simulink model "IM_ScalarCtl_adv_exercise"  (R2013b)
settings: Solver=ode45  StartTime=0.0  StopTime=3  MaxStep=1e-3  RelTol=1e-6
values from neighbouring files (symbols this model uses):
  fR = fn    (= 50)    [im_data.m]
  freq_sn = (ns-nn)/ns*fn    (= 2.33333333333)    [im_data.m]
  IactRated = In*sqrt(2)*PF    [im_data.m]
  J = jm    (= 0.0069)    [im_data.m]
  Lm = 235.0e-3    (= 0.235)    [im_data.m]
  Lr = Lm + Ldr    (= 0.24729)    [im_data.m]
  Ls = Lm + Lds    (= 0.2442)    [im_data.m]
  p = 2.0    (= 2)    [im_data.m]
  Rr = 2.32    [im_data.m]
  Rs = 3.67*1.5    (= 5.505)    [im_data.m]
  Vs0 = Un    (= 220)    [im_data.m]
libraries: powerlib_meascontrol x2, simulink x1
settings Model: Creator=unnikrishnan  LastModifiedBy=Fitim k
settings DataIOCC: SignalLoggingSaveFormat=ModelDataLogs
settings OptimizationCC: InitFltsAndDblsToZero=on
settings DebuggingCC: SaveWithParameterizedLinksMsg=none  SignalResolutionControl=TryResolveAllWithWarning  MultiTaskDSMMsg=warning  MultiTaskCondExecSysMsg=none  FcnCallInpInsideContextMsg=UseLocalSettings  StateNameClashWarn=warning
settings RTWCC: IncludeERTFirstTime=on
settings GRTTargetCC: TargetFcnLib=ansi_tfl_tmw.mat  CombineOutputUpdateFcns=off  GRTInterface=on

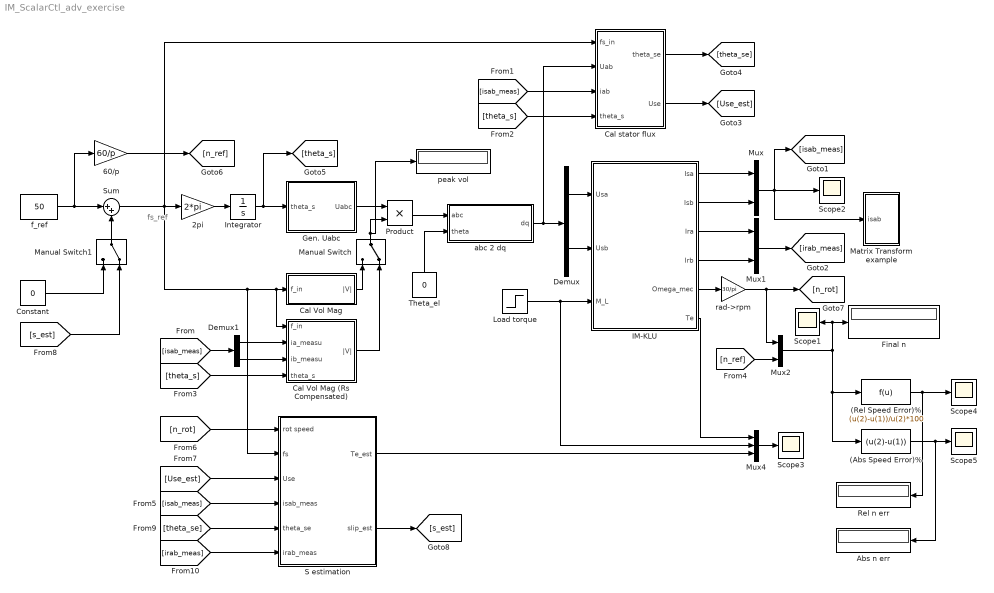
== system IM_ScalarCtl_adv_exercise ==
  note: fs_ref
  (Abs Speed Error)% : Fcn  Expr=(u(2)-u(1))
  (Rel Speed Error)% : Fcn  Expr=(u(2)-u(1))/u(2)*100
  2pi : Gain  Gain=2*pi
  60/p : Gain  Gain=60/p
  Abs n err : Display
  Cal Vol Mag : Subsystem
  Cal Vol Mag (Rs Compensated) : Subsystem
  Cal stator flux : Subsystem
  Constant : Constant  Value=0
  Demux : Demux  Outputs=2
  Demux1 : Demux  Outputs=2
  Final n : Display
  Gen. Uabc : Subsystem
  IM-KLU : Subsystem  mask(IM parameters){ms=3, pb=p, J=J, Lm=Lm, Lr=Lr, Ls=Ls, Rr=Rr, Rs=Rs}
      mask prompts: ms "number of pases"; pb "pole pairs"
  Integrator : Integrator
  Load torque : Step  After=14.6912  SampleTime=0
  Manual Switch : ManualSwitch  CurrentSetting=0
  Manual Switch1 : ManualSwitch  CurrentSetting=0
  Matrix Transform example : Subsystem
  Mux : Mux  Inputs=2
  Mux1 : Mux  Inputs=2
  Mux2 : Mux  Inputs=2
  Mux4 : Mux  Inputs=3
  Product : Product  RndMeth=Zero
  Rel n err : Display
  S estimation : Subsystem
  Scope{1..5} (5 alike) : Scope
      Scope1 settings: TimeRange=0.2881844380403459  YMin=1435  YMax=1500  SaveName=ScopeData2
      Scope2 settings: YMin=-7  YMax=7
      Scope3 settings: YMin=-2.5  YMax=25
      Scope4 settings: TimeRange=3  YMin=5.02075  YMax=5.021  SaveName=ScopeData3
      Scope5 settings: TimeRange=0.2881844380403459  YMin=0  YMax=1197.83  SaveName=ScopeData4
  Sum : Sum  Inputs=|++
  Theta_el : Constant  Value=0
  abc 2 dq : Subsystem
  f_ref : Constant  Value=50
  peak vol : Display
  rad->rpm : Gain  Gain=30/pi  SaturateOnIntegerOverflow=on  OutDataTypeStr=Inherit: Same as input  ParamDataTypeStr=Inherit: Same as input
  wires:
  f_ref/1 -> Sum/1, 60/p/1
  Constant/1 -> Manual Switch1/1
  Manual Switch1/1 -> Sum/2
  2pi/1 -> Integrator/1
  Integrator/1 -> Gen. Uabc/1(theta_s), [theta_s]
  Theta_el/1 -> abc 2 dq/2(theta)
  Product/1 -> abc 2 dq/1(abc)
  Gen. Uabc/1(Uabc) -> Product/1
  abc 2 dq/1(dq) -> Demux/1, Cal stator flux/2(Uab)
  Demux/1 -> IM-KLU/1(Usa)
  Demux/2 -> IM-KLU/2(Usb)
  Load torque/1 -> IM-KLU/3(M_L), Mux4/2
  IM-KLU/1(Isa) -> Mux/1
  IM-KLU/2(Isb) -> Mux/2
  Mux/1 -> Scope2/1, [isab_meas], Matrix Transform example/1(isab)
  IM-KLU/3(Ira) -> Mux1/1
  IM-KLU/4(Irb) -> Mux1/2
  Mux1/1 -> [irab_meas]
  Mux4/1 -> Scope3/1
  IM-KLU/6(Te) -> Mux4/1
  Mux2/1 -> (Rel Speed Error)%/1, (Abs Speed Error)%/1, Final n/1, Scope1/1
  (Rel Speed Error)%/1 -> Scope4/1, Rel n err/1
  (Abs Speed Error)%/1 -> Scope5/1, Abs n err/1
  IM-KLU/5(Omega_mec) -> rad->rpm/1
  rad->rpm/1 -> Mux2/1, [n_rot]
  Sum/1 -> 2pi/1, Cal stator flux/1(fs_in), S estimation/2(fs), Cal Vol Mag (Rs Compensated)/1(f_in), Cal Vol Mag/1(f_in)
  Demux1/1 -> Cal Vol Mag (Rs Compensated)/2(ia_measu)
  Demux1/2 -> Cal Vol Mag (Rs Compensated)/3(ib_measu)
  [isab_meas] -> Demux1/1
  Cal stator flux/1(theta_se) -> [theta_se]
  Cal stator flux/2(Use) -> [Use_est]
  [isab_meas] -> Cal stator flux/3(iab)
  [theta_s] -> Cal stator flux/4(theta_s)
  [theta_s] -> Cal Vol Mag (Rs Compensated)/4(theta_s)
  60/p/1 -> [n_ref]
  [n_ref] -> Mux2/2
  [n_rot] -> S estimation/1(rot speed)
  [Use_est] -> S estimation/3(Use)
  [isab_meas] -> S estimation/4(isab_meas)
  S estimation/2(slip_est) -> [s_est]
  [s_est] -> Manual Switch1/2
  [theta_se] -> S estimation/5(theta_se)
  [irab_meas] -> S estimation/6(irab_meas)
  Manual Switch/1 -> Product/2, peak vol/1
  Cal Vol Mag/1(|V|) -> Manual Switch/1
  Cal Vol Mag (Rs Compensated)/1(|V|) -> Manual Switch/2
  S estimation/1(Te_est) -> Mux4/3

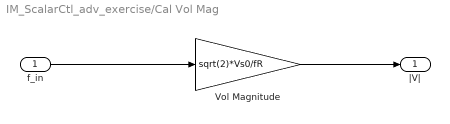
== system IM_ScalarCtl_adv_exercise/Cal Vol Mag ==
  f_in : Inport
  Vol Magnitude : Gain  Gain=sqrt(2)*Vs0/fR
  |V| : Outport
  wires:
  f_in/1 -> Vol Magnitude/1
  Vol Magnitude/1 -> |V|/1

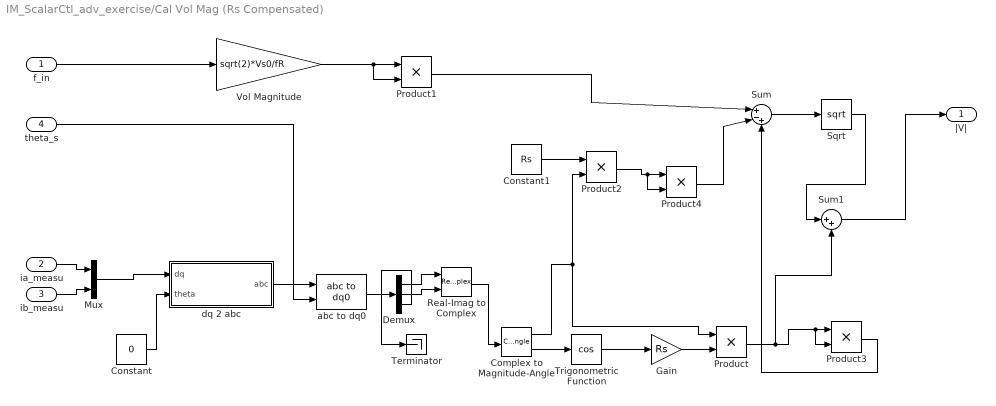
== system IM_ScalarCtl_adv_exercise/Cal Vol Mag (Rs Compensated) ==
  f_in : Inport
  ia_measu : Inport  Port=2
  ib_measu : Inport  Port=3
  theta_s : Inport  Port=4
  Complex to Magnitude-Angle : ComplexToMagnitudeAngle
  Constant : Constant  Value=0
  Constant1 : Constant  Value=Rs
  Demux : Demux  Outputs=3
  Gain : Gain  Gain=Rs
  Mux : Mux  Inputs=2
  Product{,1..4} (5 alike) : Product
  Real-Imag to Complex : RealImagToComplex
  Sqrt : Sqrt  SaturateOnIntegerOverflow=on
  Sum : Sum  Inputs=|+-+
  Sum1 : Sum  Inputs=|++
  Terminator : Terminator
  Trigonometric Function : Trigonometry  Operator=cos
  Vol Magnitude : Gain  Gain=sqrt(2)*Vs0/fR
  abc to dq0 : powerlib_meascontrol/Transformations/abc to dq0  Alignment=Aligned with phase A axis
  dq 2 abc : Subsystem
  |V| : Outport
  wires:
  ib_measu/1 -> Mux/2
  ia_measu/1 -> Mux/1
  Constant/1 -> dq 2 abc/2(theta)
  dq 2 abc/1(abc) -> abc to dq0/1
  theta_s/1 -> abc to dq0/2
  abc to dq0/1 -> Demux/1
  Demux/1 -> Real-Imag to Complex/1
  Demux/2 -> Real-Imag to Complex/2
  Real-Imag to Complex/1 -> Complex to Magnitude-Angle/1
  Demux/3 -> Terminator/1
  f_in/1 -> Vol Magnitude/1
  Complex to Magnitude-Angle/2 -> Trigonometric Function/1
  Trigonometric Function/1 -> Gain/1
  Complex to Magnitude-Angle/1 -> Product/1, Product2/2
  Vol Magnitude/1 -> Product1/2, Product1/1
  Gain/1 -> Product/2
  Constant1/1 -> Product2/1
  Product/1 -> Sum1/2, Product3/2, Product3/1
  Product3/1 -> Sum/3
  Product2/1 -> Product4/2, Product4/1
  Product1/1 -> Sum/1
  Product4/1 -> Sum/2
  Sum/1 -> Sqrt/1
  Sqrt/1 -> Sum1/1
  Sum1/1 -> |V|/1
  Mux/1 -> dq 2 abc/1(dq)

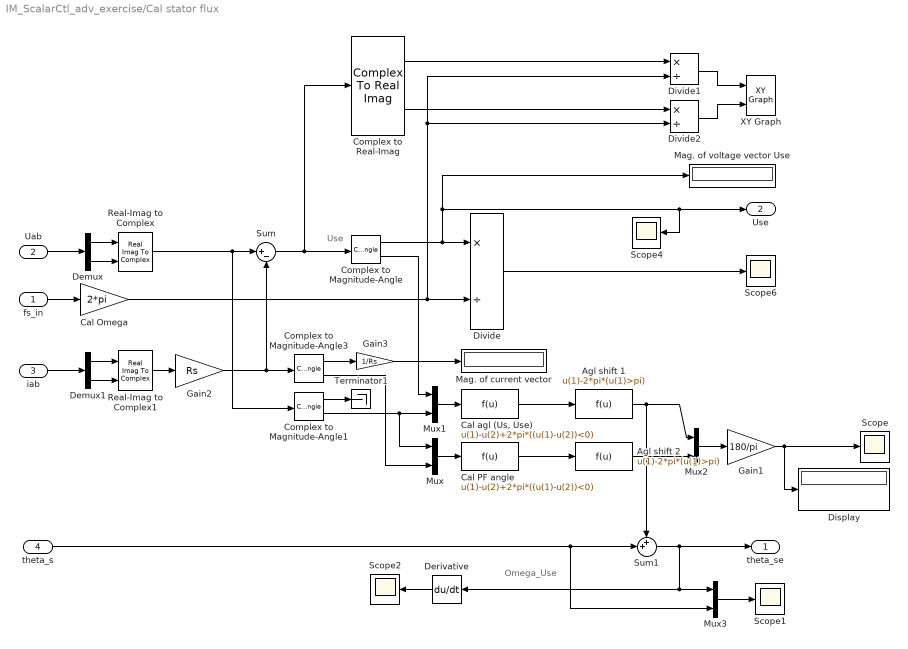
== system IM_ScalarCtl_adv_exercise/Cal stator flux ==
  note: Use
  note: Omega_Use
  fs_in : Inport
  Uab : Inport  Port=2
  iab : Inport  Port=3
  theta_s : Inport  Port=4
  Agl shift 1 : Fcn  Expr=u(1)-2*pi*(u(1)>pi)
  Agl shift 2 : Fcn  Expr=u(1)-2*pi*(u(1)>pi)
  Cal Omega : Gain  Gain=2*pi
  Cal PF angle : Fcn  Expr=u(1)-u(2)+2*pi*((u(1)-u(2))<0)
  "Cal agl (Us, Use)" : Fcn  Expr=u(1)-u(2)+2*pi*((u(1)-u(2))<0)
  Complex to Magnitude-Angle : ComplexToMagnitudeAngle
  Complex to Magnitude-Angle1 : ComplexToMagnitudeAngle
  Complex to Magnitude-Angle3 : ComplexToMagnitudeAngle
  Complex to Real-Imag : ComplexToRealImag
  Demux : Demux  Outputs=2
  Demux1 : Demux  Outputs=2
  Derivative : Derivative
  Display : Display
  Divide : Product  Inputs=*/
  Divide1 : Product  Inputs=*/
  Divide2 : Product  Inputs=*/
  Gain1 : Gain  Gain=180/pi
  Gain2 : Gain  Gain=Rs
  Gain3 : Gain  Gain=1/Rs
  Mag. of current vector : Display
  Mag. of voltage vector Use : Display
  Mux{,1..3} (4 alike) : Mux  Inputs=2
  Real-Imag to Complex : RealImagToComplex
  Real-Imag to Complex1 : RealImagToComplex
  Scope{,1..2,4,6} (5 alike) : Scope
      Scope settings: YMin=-90  YMax=140  SaveName=ScopeData9
      Scope1 settings: YMin=-90  YMax=140  SaveName=ScopeData5
      Scope2 settings: YMin=-90  YMax=140  SaveName=ScopeData10
      Scope4 settings: TimeRange=0.2881844380403459  YMin=158.3  YMax=159.4  SaveName=ScopeData21
      Scope6 settings: TimeRange=0.2881844380403459  YMin=0.940831  YMax=1.03987  SaveName=ScopeData6
  Sum : Sum  Inputs=|+-
  Sum1 : Sum  Inputs=++|
  Terminator1 : Terminator
  XY Graph : simulink/Sinks/XY Graph  xmin=-1.5  xmax=1.5  ymin=-1.5  ymax=1.5  st=-1
  theta_se : Outport
  Use : Outport  Port=2
  wires:
  Complex to Magnitude-Angle/1 -> Divide/1, Mag. of voltage vector Use/1, Use/1, Scope4/1
  Cal Omega/1 -> Divide/2, Divide2/2, Divide1/2
  fs_in/1 -> Cal Omega/1
  Complex to Real-Imag/1 -> Divide1/1
  Complex to Real-Imag/2 -> Divide2/1
  Divide1/1 -> XY Graph/1
  Divide2/1 -> XY Graph/2
  Mux/1 -> Cal PF angle/1
  Gain1/1 -> Display/1, Scope/1
  Mux1/1 -> "Cal agl (Us, Use)"/1
  Mux2/1 -> Gain1/1
  Cal PF angle/1 -> Agl shift 2/1
  "Cal agl (Us, Use)"/1 -> Agl shift 1/1
  Divide/1 -> Scope6/1
  Gain2/1 -> Sum/2, Complex to Magnitude-Angle3/1
  Sum/1 -> Complex to Magnitude-Angle/1, Complex to Real-Imag/1
  Complex to Magnitude-Angle1/1 -> Terminator1/1
  Complex to Magnitude-Angle1/2 -> Mux/1, Mux1/2
  Complex to Magnitude-Angle3/1 -> Gain3/1
  Complex to Magnitude-Angle3/2 -> Mux/2
  Agl shift 1/1 -> Mux2/1, Sum1/1
  Agl shift 2/1 -> Mux2/2
  theta_s/1 -> Sum1/2, Mux3/2
  Sum1/1 -> theta_se/1, Mux3/1, Derivative/1
  Uab/1 -> Demux/1
  Demux/1 -> Real-Imag to Complex/1
  Demux/2 -> Real-Imag to Complex/2
  Real-Imag to Complex/1 -> Sum/1, Complex to Magnitude-Angle1/1
  Demux1/1 -> Real-Imag to Complex1/1
  iab/1 -> Demux1/1
  Real-Imag to Complex1/1 -> Gain2/1
  Demux1/2 -> Real-Imag to Complex1/2
  Mux3/1 -> Scope1/1
  Complex to Magnitude-Angle/2 -> Mux1/1
  Derivative/1 -> Scope2/1
  Gain3/1 -> Mag. of current vector/1

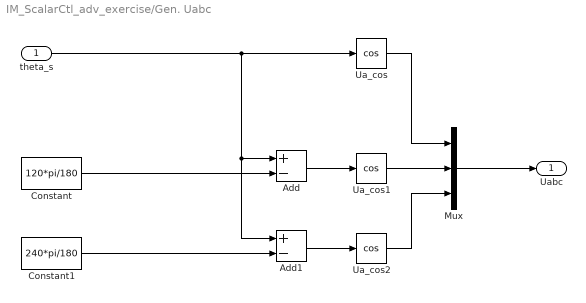
== system IM_ScalarCtl_adv_exercise/Gen. Uabc ==
  theta_s : Inport
  Add : Sum  Inputs=+-
  Add1 : Sum  Inputs=+-
  Constant : Constant  Value=120*pi/180
  Constant1 : Constant  Value=240*pi/180
  Mux : Mux  Inputs=3
  Ua_cos : Trigonometry  Operator=cos
  Ua_cos1 : Trigonometry  Operator=cos
  Ua_cos2 : Trigonometry  Operator=cos
  Uabc : Outport
  wires:
  Constant/1 -> Add/2
  Constant1/1 -> Add1/2
  theta_s/1 -> Ua_cos/1, Add/1, Add1/1
  Add/1 -> Ua_cos1/1
  Add1/1 -> Ua_cos2/1
  Ua_cos/1 -> Mux/1
  Ua_cos1/1 -> Mux/2
  Ua_cos2/1 -> Mux/3
  Mux/1 -> Uabc/1

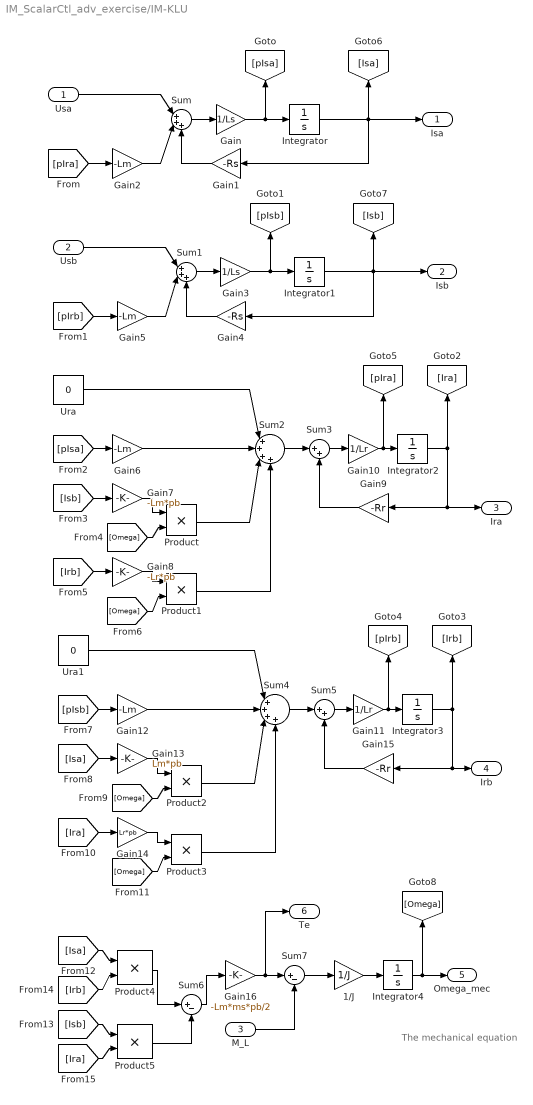
== system IM_ScalarCtl_adv_exercise/IM-KLU ==
  note: The mechanical equation
  Usa : Inport
  Usb : Inport  Port=2
  M_L : Inport  Port=3
  1/J : Gain  Gain=1/J  SaturateOnIntegerOverflow=on  OutDataTypeStr=Inherit: Same as input  ParamDataTypeStr=Inherit: Same as input
  Gain : Gain  Gain=1/Ls  SaturateOnIntegerOverflow=on  OutDataTypeStr=Inherit: Same as input  ParamDataTypeStr=Inherit: Same as input
  Gain1 : Gain  Gain=-Rs  SaturateOnIntegerOverflow=on  OutDataTypeStr=Inherit: Same as input  ParamDataTypeStr=Inherit: Same as input
  Gain10 : Gain  Gain=1/Lr  SaturateOnIntegerOverflow=on  OutDataTypeStr=Inherit: Same as input  ParamDataTypeStr=Inherit: Same as input
  Gain11 : Gain  Gain=1/Lr  SaturateOnIntegerOverflow=on  OutDataTypeStr=Inherit: Same as input  ParamDataTypeStr=Inherit: Same as input
  Gain{2,5..6,12} (4 alike) : Gain  Gain=-Lm  SaturateOnIntegerOverflow=on  OutDataTypeStr=Inherit: Same as input  ParamDataTypeStr=Inherit: Same as input
  Gain13 : Gain  Gain=Lm*pb  SaturateOnIntegerOverflow=on  OutDataTypeStr=Inherit: Same as input  ParamDataTypeStr=Inherit: Same as input
  Gain14 : Gain  Gain=Lr*pb  SaturateOnIntegerOverflow=on  OutDataTypeStr=Inherit: Same as input  ParamDataTypeStr=Inherit: Same as input
  Gain15 : Gain  Gain=-Rr  SaturateOnIntegerOverflow=on  OutDataTypeStr=Inherit: Same as input  ParamDataTypeStr=Inherit: Same as input
  Gain16 : Gain  Gain=-Lm*ms*pb/2  SaturateOnIntegerOverflow=on  OutDataTypeStr=Inherit: Same as input  ParamDataTypeStr=Inherit: Same as input
  Gain3 : Gain  Gain=1/Ls  SaturateOnIntegerOverflow=on  OutDataTypeStr=Inherit: Same as input  ParamDataTypeStr=Inherit: Same as input
  Gain4 : Gain  Gain=-Rs  SaturateOnIntegerOverflow=on  OutDataTypeStr=Inherit: Same as input  ParamDataTypeStr=Inherit: Same as input
  Gain7 : Gain  Gain=-Lm*pb  SaturateOnIntegerOverflow=on  OutDataTypeStr=Inherit: Same as input  ParamDataTypeStr=Inherit: Same as input
  Gain8 : Gain  Gain=-Lr*pb  SaturateOnIntegerOverflow=on  OutDataTypeStr=Inherit: Same as input  ParamDataTypeStr=Inherit: Same as input
  Gain9 : Gain  Gain=-Rr  SaturateOnIntegerOverflow=on  OutDataTypeStr=Inherit: Same as input  ParamDataTypeStr=Inherit: Same as input
  Integrator{,1..4} (5 alike) : Integrator
  Product{,1..5} (6 alike) : Product  SaturateOnIntegerOverflow=on  RndMeth=Zero  InputSameDT=on  OutDataTypeStr=Inherit: Same as first input
  Sum : Sum  Inputs=|+++  SaturateOnIntegerOverflow=on  InputSameDT=on  OutDataTypeStr=Inherit: Same as first input
  Sum1 : Sum  Inputs=|+++  SaturateOnIntegerOverflow=on  InputSameDT=on  OutDataTypeStr=Inherit: Same as first input
  Sum2 : Sum  Inputs=|++++  SaturateOnIntegerOverflow=on  InputSameDT=on  OutDataTypeStr=Inherit: Same as first input
  Sum3 : Sum  Inputs=|++  SaturateOnIntegerOverflow=on  InputSameDT=on  OutDataTypeStr=Inherit: Same as first input
  Sum4 : Sum  Inputs=|++++  SaturateOnIntegerOverflow=on  InputSameDT=on  OutDataTypeStr=Inherit: Same as first input
  Sum5 : Sum  Inputs=|++  SaturateOnIntegerOverflow=on  InputSameDT=on  OutDataTypeStr=Inherit: Same as first input
  Sum6 : Sum  Inputs=|+-  SaturateOnIntegerOverflow=on  InputSameDT=on  OutDataTypeStr=Inherit: Same as first input
  Sum7 : Sum  Inputs=|+-  SaturateOnIntegerOverflow=on  InputSameDT=on  OutDataTypeStr=Inherit: Same as first input
  Ura : Constant  Value=0
  Ura1 : Constant  Value=0
  Isa : Outport
  Isb : Outport  Port=2
  Ira : Outport  Port=3
  Irb : Outport  Port=4
  Omega_mec : Outport  Port=5
  Te : Outport  Port=6
  wires:
  Usa/1 -> Sum/1
  Gain1/1 -> Sum/3
  Sum/1 -> Gain/1
  Integrator/1 -> Isa/1, Gain1/1, [Isa]
  Gain2/1 -> Sum/2
  [pIra] -> Gain2/1
  Gain/1 -> Integrator/1, [pIsa]
  Usb/1 -> Sum1/1
  Gain4/1 -> Sum1/3
  Sum1/1 -> Gain3/1
  Integrator1/1 -> Isb/1, Gain4/1, [Isb]
  Gain5/1 -> Sum1/2
  [pIrb] -> Gain5/1
  Gain3/1 -> Integrator1/1, [pIsb]
  Ura/1 -> Sum2/1
  [pIsa] -> Gain6/1
  Gain6/1 -> Sum2/2
  [Isb] -> Gain7/1
  [Omega] -> Product/2
  Product/1 -> Sum2/3
  [Irb] -> Gain8/1
  Gain8/1 -> Product1/1
  Product1/1 -> Sum2/4
  Sum2/1 -> Sum3/1
  Sum3/1 -> Gain10/1
  Gain9/1 -> Sum3/2
  Integrator2/1 -> [Ira], Gain9/1, Ira/1
  Ura1/1 -> Sum4/1
  [pIsb] -> Gain12/1
  Gain12/1 -> Sum4/2
  [Isa] -> Gain13/1
  [Omega] -> Product2/2
  Product2/1 -> Sum4/3
  [Ira] -> Gain14/1
  Gain14/1 -> Product3/1
  Product3/1 -> Sum4/4
  Sum4/1 -> Sum5/1
  Sum5/1 -> Gain11/1
  Gain15/1 -> Sum5/2
  Integrator3/1 -> [Irb], Gain15/1, Irb/1
  Gain11/1 -> Integrator3/1, [pIrb]
  Sum6/1 -> Gain16/1
  Gain16/1 -> Sum7/1, Te/1
  M_L/1 -> Sum7/2
  Sum7/1 -> 1/J/1
  1/J/1 -> Integrator4/1
  [Isa] -> Product4/1
  [Isb] -> Product5/1
  [Ira] -> Product5/2
  Integrator4/1 -> [Omega], Omega_mec/1
  [Irb] -> Product4/2
  [Omega] -> Product3/2
  Gain13/1 -> Product2/1
  [Omega] -> Product1/2
  Gain7/1 -> Product/1
  Gain10/1 -> Integrator2/1, [pIra]
  Product4/1 -> Sum6/1
  Product5/1 -> Sum6/2

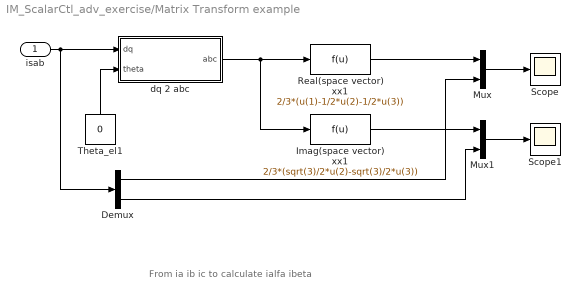
== system IM_ScalarCtl_adv_exercise/Matrix Transform example ==
  note: From ia ib ic to calculate ialfa ibeta
  isab : Inport
  Demux : Demux  Outputs=2
  Imag(space vector) xx1 : Fcn  Expr=2/3*(sqrt(3)/2*u(2)-sqrt(3)/2*u(3))
  Mux : Mux  Inputs=2
  Mux1 : Mux  Inputs=2
  Real(space vector) xx1 : Fcn  Expr=2/3*(u(1)-1/2*u(2)-1/2*u(3))
  Scope : Scope
      settings: SaveName=ScopeData7
  Scope1 : Scope
      settings: SaveName=ScopeData8
  Theta_el1 : Constant  Value=0
  dq 2 abc : Subsystem
  wires:
  Theta_el1/1 -> dq 2 abc/2(theta)
  isab/1 -> dq 2 abc/1(dq), Demux/1
  dq 2 abc/1(abc) -> Real(space vector) xx1/1, Imag(space vector) xx1/1
  Real(space vector) xx1/1 -> Mux/1
  Demux/1 -> Mux/2
  Imag(space vector) xx1/1 -> Mux1/1
  Demux/2 -> Mux1/2
  Mux/1 -> Scope/1
  Mux1/1 -> Scope1/1

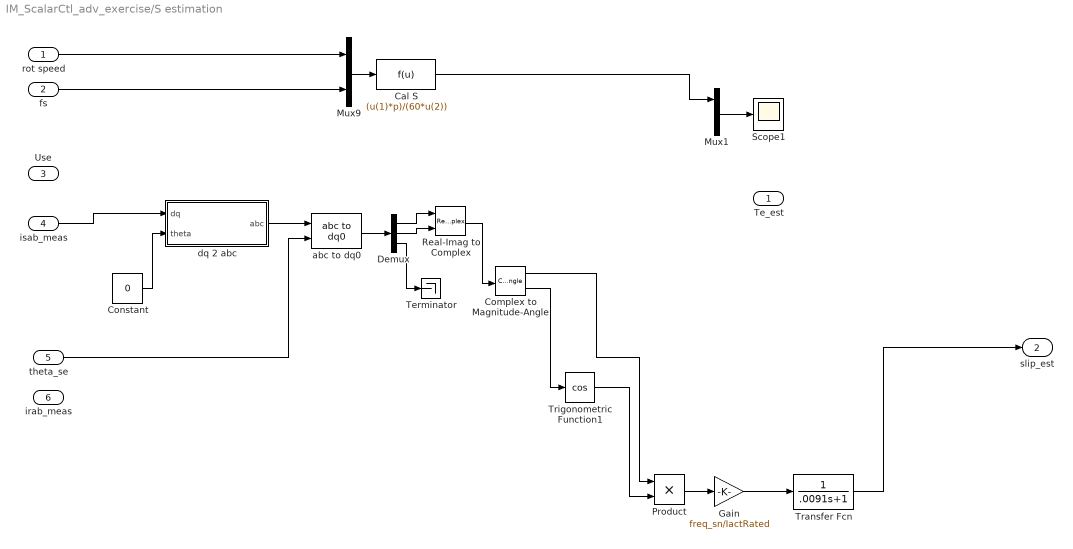
== system IM_ScalarCtl_adv_exercise/S estimation ==
  rot speed : Inport
  fs : Inport  Port=2
  Use : Inport  Port=3
  isab_meas : Inport  Port=4
  theta_se : Inport  Port=5
  irab_meas : Inport  Port=6
  Cal S : Fcn  Expr=(u(1)*p)/(60*u(2))
  Complex to Magnitude-Angle : ComplexToMagnitudeAngle
  Constant : Constant  Value=0
  Demux : Demux  Outputs=3
  Gain : Gain  Gain=freq_sn/IactRated
  Mux1 : Mux  Inputs=2
  Mux9 : Mux  Inputs=2
  Product : Product
  Real-Imag to Complex : RealImagToComplex
  Scope1 : Scope
      settings: YMin=0  YMax=1.05  SaveName=ScopeData11
  Terminator : Terminator
  Transfer Fcn : TransferFcn  Denominator=[.0091 1]
  Trigonometric Function1 : Trigonometry  Operator=cos
  abc to dq0 : powerlib_meascontrol/Transformations/abc to dq0  Alignment=Aligned with phase A axis
  dq 2 abc : Subsystem
  Te_est : Outport
  slip_est : Outport  Port=2
  wires:
  Mux9/1 -> Cal S/1
  rot speed/1 -> Mux9/1
  fs/1 -> Mux9/2
  Cal S/1 -> Mux1/1
  Mux1/1 -> Scope1/1
  Constant/1 -> dq 2 abc/2(theta)
  dq 2 abc/1(abc) -> abc to dq0/1
  abc to dq0/1 -> Demux/1
  Demux/1 -> Real-Imag to Complex/1
  Demux/2 -> Real-Imag to Complex/2
  Real-Imag to Complex/1 -> Complex to Magnitude-Angle/1
  Demux/3 -> Terminator/1
  isab_meas/1 -> dq 2 abc/1(dq)
  Complex to Magnitude-Angle/2 -> Trigonometric Function1/1
  Complex to Magnitude-Angle/1 -> Product/1
  Trigonometric Function1/1 -> Product/2
  Product/1 -> Gain/1
  Gain/1 -> Transfer Fcn/1
  theta_se/1 -> abc to dq0/2
  Transfer Fcn/1 -> slip_est/1

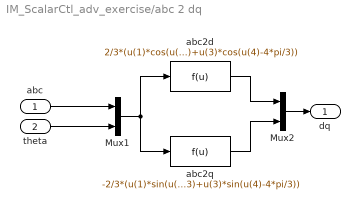
== system IM_ScalarCtl_adv_exercise/abc 2 dq ==
  abc : Inport
  theta : Inport  Port=2
  Mux1 : Mux  Inputs=2
  Mux2 : Mux  Inputs=2
  abc2d : Fcn  Expr=2/3*(u(1)*cos(u(4))+u(2)*cos(u(4)-2*pi/3)+u(3)*cos(u(4)-4*pi/3))
  abc2q : Fcn  Expr=-2/3*(u(1)*sin(u(4))+u(2)*sin(u(4)-2*pi/3)+u(3)*sin(u(4)-4*pi/3))
  dq : Outport
  wires:
  abc/1 -> Mux1/1
  theta/1 -> Mux1/2
  Mux1/1 -> abc2d/1, abc2q/1
  abc2d/1 -> Mux2/1
  abc2q/1 -> Mux2/2
  Mux2/1 -> dq/1

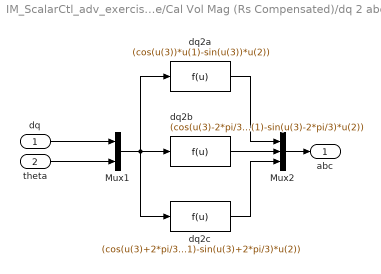
== system IM_ScalarCtl_adv_exercise/Cal Vol Mag (Rs Compensated)/dq 2 abc ==
  dq : Inport
  theta : Inport  Port=2
  Mux1 : Mux  Inputs=2
  Mux2 : Mux  Inputs=3
  dq2a : Fcn  Expr=(cos(u(3))*u(1)-sin(u(3))*u(2))
  dq2b : Fcn  Expr=(cos(u(3)-2*pi/3)*u(1)-sin(u(3)-2*pi/3)*u(2))
  dq2c : Fcn  Expr=(cos(u(3)+2*pi/3)*u(1)-sin(u(3)+2*pi/3)*u(2))
  abc : Outport
  wires:
  Mux2/1 -> abc/1
  dq2b/1 -> Mux2/2
  dq2a/1 -> Mux2/1
  Mux1/1 -> dq2a/1, dq2c/1, dq2b/1
  theta/1 -> Mux1/2
  dq/1 -> Mux1/1
  dq2c/1 -> Mux2/3

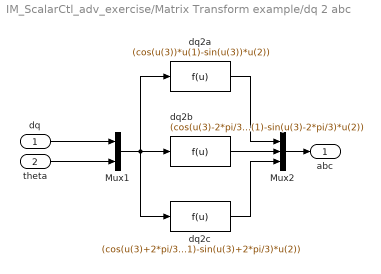
== system IM_ScalarCtl_adv_exercise/Matrix Transform example/dq 2 abc ==
  dq : Inport
  theta : Inport  Port=2
  Mux1 : Mux  Inputs=2
  Mux2 : Mux  Inputs=3
  dq2a : Fcn  Expr=(cos(u(3))*u(1)-sin(u(3))*u(2))
  dq2b : Fcn  Expr=(cos(u(3)-2*pi/3)*u(1)-sin(u(3)-2*pi/3)*u(2))
  dq2c : Fcn  Expr=(cos(u(3)+2*pi/3)*u(1)-sin(u(3)+2*pi/3)*u(2))
  abc : Outport
  wires:
  Mux2/1 -> abc/1
  dq2b/1 -> Mux2/2
  dq2a/1 -> Mux2/1
  Mux1/1 -> dq2a/1, dq2c/1, dq2b/1
  theta/1 -> Mux1/2
  dq/1 -> Mux1/1
  dq2c/1 -> Mux2/3

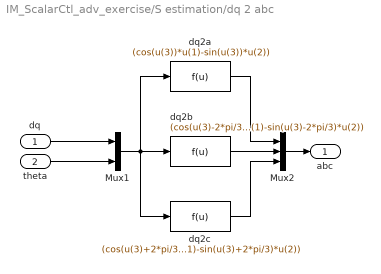
== system IM_ScalarCtl_adv_exercise/S estimation/dq 2 abc ==
  dq : Inport
  theta : Inport  Port=2
  Mux1 : Mux  Inputs=2
  Mux2 : Mux  Inputs=3
  dq2a : Fcn  Expr=(cos(u(3))*u(1)-sin(u(3))*u(2))
  dq2b : Fcn  Expr=(cos(u(3)-2*pi/3)*u(1)-sin(u(3)-2*pi/3)*u(2))
  dq2c : Fcn  Expr=(cos(u(3)+2*pi/3)*u(1)-sin(u(3)+2*pi/3)*u(2))
  abc : Outport
  wires:
  Mux2/1 -> abc/1
  dq2b/1 -> Mux2/2
  dq2a/1 -> Mux2/1
  Mux1/1 -> dq2a/1, dq2c/1, dq2b/1
  theta/1 -> Mux1/2
  dq/1 -> Mux1/1
  dq2c/1 -> Mux2/3
